simulink model "sudoku_test"  (R2018b)
settings: Solver=FixedStepDiscrete  StartTime=0.0  StopTime=1  FixedStep=1  RelTol=1e-3
libraries: sudoku_lib x7
settings Model: Creator=F074018  LastModifiedBy=F074018
settings DebuggingCC: InheritedTsInSrcMsg=none

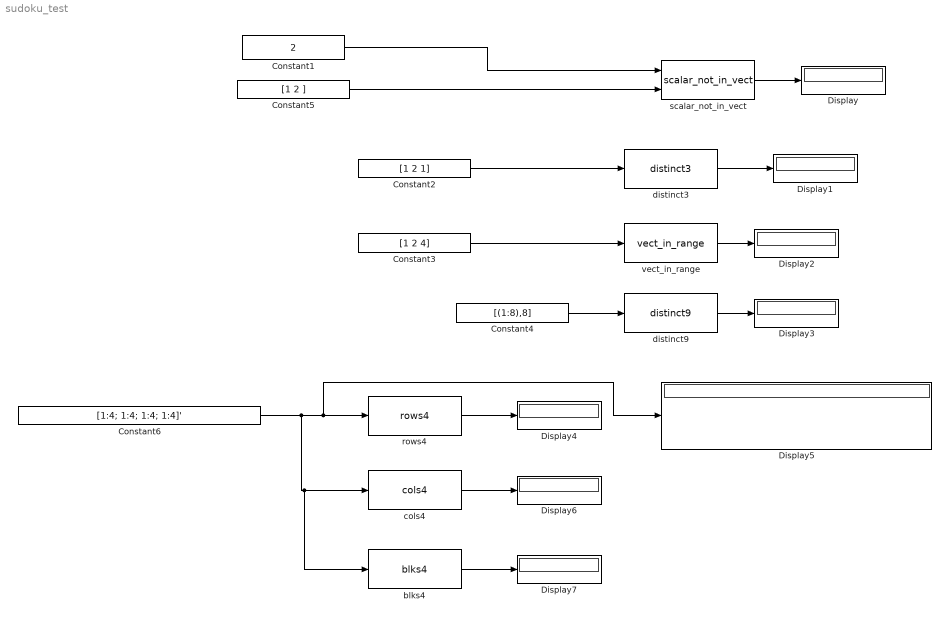
== system sudoku_test ==
  Constant1 : Constant  Value=2  OutDataTypeStr=uint8
  Constant2 : Constant  Value=[1 2 1]  OutDataTypeStr=uint8
  Constant3 : Constant  Value=[1 2 4]  OutDataTypeStr=uint8
  Constant4 : Constant  Value=[(1:8),8]  OutDataTypeStr=uint8
  Constant5 : Constant  Value=[1 2 ]  OutDataTypeStr=uint8
  Constant6 : Constant  Value=[1:4; 1:4; 1:4; 1:4]'  OutDataTypeStr=uint8
  Display{,1..7} (8 alike) : Display
  blks4 : sudoku_lib/blks4  SystemSampleTime=-1
  cols4 : sudoku_lib/cols4  SystemSampleTime=-1
  distinct3 : sudoku_lib/distinct3  SystemSampleTime=-1
  distinct9 : sudoku_lib/distinct9  SystemSampleTime=-1
  rows4 : sudoku_lib/rows4  SystemSampleTime=-1
  scalar_not_in_vect : sudoku_lib/scalar_not_in_vect  SystemSampleTime=-1
  vect_in_range : sudoku_lib/vect_in_range  SystemSampleTime=-1
  wires:
  Constant1/1 -> scalar_not_in_vect/1
  Constant5/1 -> scalar_not_in_vect/2
  scalar_not_in_vect/1 -> Display/1
  Constant2/1 -> distinct3/1
  distinct3/1 -> Display1/1
  vect_in_range/1 -> Display2/1
  Constant3/1 -> vect_in_range/1
  distinct9/1 -> Display3/1
  Constant4/1 -> distinct9/1
  rows4/1 -> Display4/1
  Constant6/1 -> blks4/1, cols4/1, Display5/1, rows4/1
  cols4/1 -> Display6/1
  blks4/1 -> Display7/1
